simulink model "gatito"  (R2012b)
settings: Solver=ode45  StartTime=0.0  StopTime=100.0  RelTol=1e-3
undefined symbols (not defined in the file): gato
libraries: simulink x1
settings Model: Creator=Daniel  LastModifiedBy=Daniel

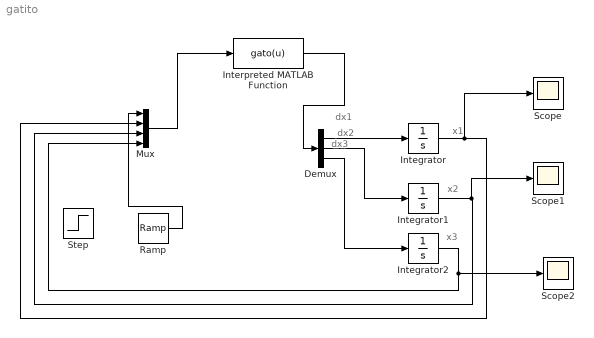
== system gatito ==
  note: x3
  note: x2
  note: x1
  note: dx3
  note: dx2
  note: dx1
  Demux : Demux  Outputs=3
  Integrator : Integrator
  Integrator1 : Integrator
  Integrator2 : Integrator
  Interpreted MATLAB Function : MATLABFcn  MATLABFcn=gato(u)
  Mux : Mux
  Ramp : simulink/Sources/Ramp  slope=1  start=0  X0=0
  Scope : Scope
  Scope1 : Scope
  Scope2 : Scope
      settings: SaveName=ScopeData2
  Step : Step  SampleTime=0
  wires:
  Interpreted MATLAB Function/1 -> Demux/1
  Mux/1 -> Interpreted MATLAB Function/1
  Demux/1 -> Integrator/1
  Demux/2 -> Integrator1/1
  Demux/3 -> Integrator2/1
  Integrator2/1 -> Scope2/1, Mux/4
  Integrator1/1 -> Scope1/1, Mux/3
  Integrator/1 -> Scope/1, Mux/2
  Ramp/1 -> Mux/1
